simulink model "laba_4"  (Simulink 9.2)
settings: Solver=FixedStepAuto  StartTime=0.0  StopTime=10  FixedStep=0.0001  RelTol=1e-3  EnableMultiTasking=on
settings Model: Creator=student  LastModifiedBy=murad  SnapshotInterval=100
settings OptimizationCC: ExpressionDepthLimit=2147483647
settings DebuggingCC: SolverPrmCheckMsg=warning

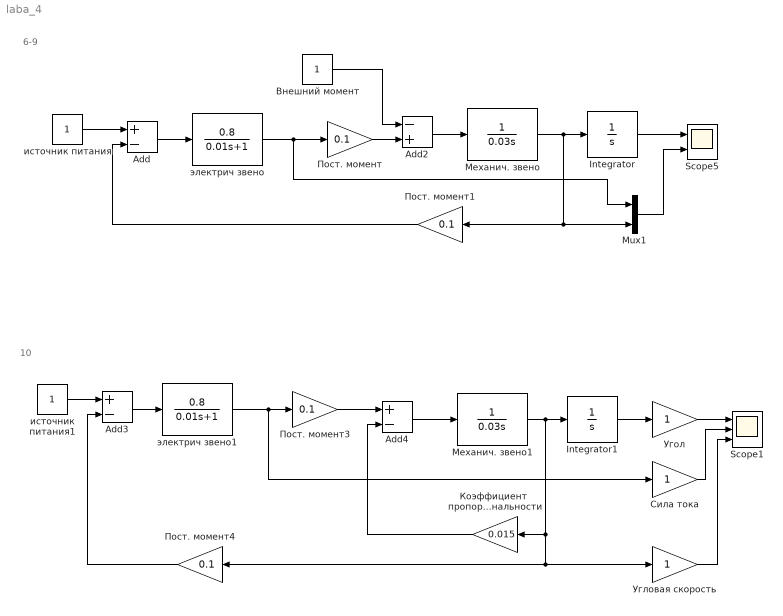
== system laba_4 ==
  note: 6-9
  note: 10
  Add : Sum  Inputs=+-
  Add2 : Sum  Inputs=-+
  Add3 : Sum  Inputs=+-
  Add4 : Sum  Inputs=+-
  Integrator : Integrator
  Integrator1 : Integrator
  Mux1 : Mux  Inputs=2
  Scope1 : Scope  NumInputPorts=3
  Scope5 : Scope  NumInputPorts=2
  Внешний момент : Constant
  Коэффициент  пропорциональности : Gain  Gain=0.015
  Механич. звено : TransferFcn  Denominator=[0.03 0]
  Механич. звено1 : TransferFcn  Denominator=[0.03 0]
  Пост. момент{,1,3..4} (4 alike) : Gain  Gain=0.1
  Сила тока : Gain
  Угловая скорость : Gain
  "Угол " : Gain
  источник питания : Constant
  источник питания1 : Constant
  электрич звено : TransferFcn  Numerator=[0.8]  Denominator=[0.01 1]
  электрич звено1 : TransferFcn  Numerator=[0.8]  Denominator=[0.01 1]
  wires:
  источник питания/1 -> Add/1
  Add/1 -> электрич звено/1
  электрич звено/1 -> Mux1/1, Пост. момент/1
  Механич. звено/1 -> Integrator/1, Mux1/2, Пост. момент1/1
  Пост. момент1/1 -> Add/2
  Mux1/1 -> Scope5/2
  Integrator/1 -> Scope5/1
  Add3/1 -> электрич звено1/1
  Механич. звено1/1 -> Коэффициент  пропорциональности/1, Угловая скорость/1, Пост. момент4/1, Integrator1/1
  электрич звено1/1 -> Сила тока/1, Пост. момент3/1
  Пост. момент4/1 -> Add3/2
  Add4/1 -> Механич. звено1/1
  источник питания1/1 -> Add3/1
  Пост. момент3/1 -> Add4/1
  Коэффициент  пропорциональности/1 -> Add4/2
  Add2/1 -> Механич. звено/1
  Пост. момент/1 -> Add2/2
  Внешний момент/1 -> Add2/1
  Сила тока/1 -> Scope1/2
  Угловая скорость/1 -> Scope1/3
  Integrator1/1 -> "Угол "/1
  "Угол "/1 -> Scope1/1
